simulink model "ironCub"  (Simulink 8.6)
settings: Solver=FixedStepAuto  StartTime=0.0  StopTime=config.simulationTime  FixedStep=config.Ts  RelTol=1e-3
InitFcn:
  | cd(fileparts(which(bdroot)));
  | initIronCub;
StopFcn:
  | visualizer_demo(time.Data,state.Data,config,desired_x_dx_ddx_dddx_CoM,jetsIntensitiesByWeight);
values from neighbouring files (symbols this model uses):
  config = struct    [initIronCub.m]
  ROBOT_DOF = config.ndof    [initIronCub.m]
libraries: WBToolboxLibrary x99
(part 1 of 2)
settings Model: Creator=DanielePucci  LastModifiedBy=DanielePucci
settings DataIOCC: SaveFormat=Dataset  SignalLoggingSaveFormat=Dataset
settings OptimizationCC: ExpressionDepthLimit=128
settings DebuggingCC: UnderspecifiedInitializationDetection=Simplified  MergeDetectMultiDrivingBlocksExec=error  SolverPrmCheckMsg=none  FcnCallInpInsideContextMsg=EnableAllAsError  StateNameClashWarn=none
settings HardwareCC: ProdBitPerPointer=64  ProdLargestAtomicFloat=Float  ProdIntDivRoundTo=Zero  ProdEndianess=LittleEndian  ProdWordSize=64  ProdHWDeviceType=Intel->x86-64 (Windows64)
settings GRTTargetCC: GeneratePreprocessorConditionals=Use local settings  CombineOutputUpdateFcns=on  GRTInterface=off
settings ConfigComp: CovModelRefEnable=off

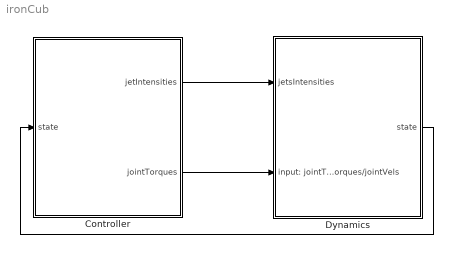
== system ironCub ==
  Controller : Subsystem
  Dynamics : Subsystem
  wires:
  Controller/1(jetIntensities) -> Dynamics/1(jetsIntensities)
  Controller/2(jointTorques) -> Dynamics/2(input: jointTorques/jointVels)
  Dynamics/1(state) -> Controller/1(state)

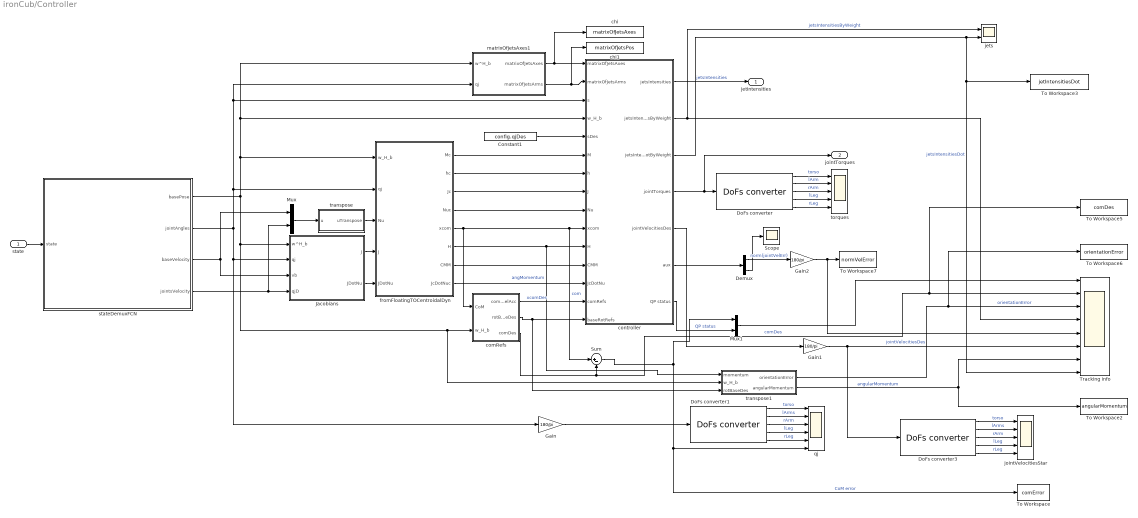
== system ironCub/Controller ==
  state : Inport
  Constant1 : Constant  Value=config.qjDes
  Demux : Demux  Outputs=2
  DoFs converter : WBToolboxLibrary/Utilities/DoFs converter  yarp2WBIOption=From WBI to YARP  robotName=WBT_robotName  localName=WBT_modelName  wbiFile=WBT_wbiFilename  wbiList=WBT_wbiList
  DoFs converter1 : WBToolboxLibrary/Utilities/DoFs converter  yarp2WBIOption=From WBI to YARP  robotName=WBT_robotName  localName=WBT_modelName  wbiFile=WBT_wbiFilename  wbiList=WBT_wbiList
  DoFs converter3 : WBToolboxLibrary/Utilities/DoFs converter  yarp2WBIOption=From WBI to YARP  robotName=WBT_robotName  localName=WBT_modelName  wbiFile=WBT_wbiFilename  wbiList=WBT_wbiList
  Gain : Gain  Gain=180/pi
  Gain1 : Gain  Gain=180/pi
  Gain2 : Gain  Gain=180/pi
  Jacobians : Subsystem
  Mux : Mux  Inputs=2
  Mux1 : Mux  Inputs=2
  Scope : Scope
  Sum : Sum  Inputs=|+-
  To Workspace : ToWorkspace  VariableName=comError  SaveFormat=Timeseries  SampleTime=-1
  To Workspace2 : ToWorkspace  VariableName=angularMomentum  SaveFormat=Timeseries  SampleTime=-1
  To Workspace3 : ToWorkspace  VariableName=jetIntensitiesDot  SaveFormat=Timeseries  SampleTime=-1
  To Workspace5 : ToWorkspace  VariableName=comDes  SaveFormat=Timeseries  SampleTime=-1
  To Workspace6 : ToWorkspace  VariableName=orientationError  SaveFormat=Timeseries  SampleTime=-1
  To Workspace7 : ToWorkspace  VariableName=normVelError  SaveFormat=Timeseries  SampleTime=-1
  Tracking info : Scope  NumInputPorts=8
  chi : ToWorkspace  VariableName=matrixOfJetsAxes  SaveFormat=Timeseries  SampleTime=-1
  chi1 : ToWorkspace  VariableName=matrixOfJetsPos  SaveFormat=Timeseries  SampleTime=-1
  comRefs : Subsystem
  controller : Subsystem
  fromFloatingTOCentroidalDyn : Subsystem
  jets : Scope  NumInputPorts=2
  jointVelocitiesStar : Scope  NumInputPorts=5
  matrixOfJetsAxes1 : Subsystem
  qj : Scope  NumInputPorts=6
  stateDemuxFCN : MATLAB Function  TreatAsAtomicUnit=on
  torques : Scope  NumInputPorts=5
  transpose : MATLAB Function  TreatAsAtomicUnit=on
  transpose1 : MATLAB Function  TreatAsAtomicUnit=on
  jetIntensities : Outport
  jointTorques : Outport  Port=2
  wires:
  state/1 -> stateDemuxFCN/1(state)
  stateDemuxFCN/4(jointsVelocity) -> Mux/2, Jacobians/4(qjD)
  stateDemuxFCN/2(jointAngles) -> Gain/1, Jacobians/2(qj), matrixOfJetsAxes1/2(qj), controller/3(s), fromFloatingTOCentroidalDyn/2(qj)
  stateDemuxFCN/1(basePose) -> controller/4(w_H_b), matrixOfJetsAxes1/1(w^H_b), fromFloatingTOCentroidalDyn/1(w_H_b), transpose1/2(w_H_b), comRefs/2(w_H_b), Jacobians/1(w^H_b)
  Jacobians/1(J) -> fromFloatingTOCentroidalDyn/4(J)
  matrixOfJetsAxes1/1(matrixOfJetsAxes) -> chi/1, controller/1(matrixOfJetsAxes)
  stateDemuxFCN/3(baseVelocity) -> Mux/1, Jacobians/3(vb)
  fromFloatingTOCentroidalDyn/1(Mc) -> controller/6(M)
  fromFloatingTOCentroidalDyn/2("hc ") -> controller/7(h)
  fromFloatingTOCentroidalDyn/3(Jc) -> controller/8(J)
  fromFloatingTOCentroidalDyn/4(Nuc) -> controller/9(Nu)
  fromFloatingTOCentroidalDyn/5(xcom) -> Sum/1, controller/10(xcom), comRefs/1(CoM)  "com"
  controller/4(jointTorques) -> DoFs converter/1, jointTorques/1
  controller/1(jetsIntensities) -> jetIntensities/1  "jetsIntensities"
  Constant1/1 -> controller/5(sDes)
  comRefs/1(comDesPosVelAcc) -> controller/14(comRefs)  "xcomDes"
  Sum/1 -> Mux1/1, qj/6, To Workspace/1  "CoM error"
  DoFs converter1/3 -> qj/3  "rArm"
  DoFs converter1/1 -> qj/1  "torso"
  DoFs converter1/4 -> qj/4  "lLeg"
  DoFs converter1/2 -> qj/2  "lArms"
  DoFs converter1/5 -> qj/5  "rLeg"
  DoFs converter/3 -> torques/3  "rArm"
  DoFs converter/1 -> torques/1  "torso"
  DoFs converter/4 -> torques/4  "lLeg"
  DoFs converter/2 -> torques/2  "lArm"
  DoFs converter/5 -> torques/5  "rLeg"
  Mux/1 -> transpose/1(u)
  transpose/1(uTranspose) -> fromFloatingTOCentroidalDyn/3(Nu)
  Jacobians/2(JDotNu) -> fromFloatingTOCentroidalDyn/5(JDotNu)
  fromFloatingTOCentroidalDyn/8(JcDotNuc) -> controller/13(JcDotNu)
  matrixOfJetsAxes1/2(matrixOfJetsArms) -> chi1/1, controller/2(matrixOfJetsArms)
  fromFloatingTOCentroidalDyn/6(H) -> transpose1/1(momentum), controller/11(H)  "angMomentum"
  fromFloatingTOCentroidalDyn/7(CMM) -> controller/12(CMM)
  Gain/1 -> DoFs converter1/1
  controller/6(aux) -> Demux/1
  Demux/1 -> Gain2/1  "norm(jointVelErr)"
  controller/5(jointVelocitiesDes) -> Gain1/1
  transpose1/1(orientationError) -> To Workspace6/1, Tracking info/3  "orientationError"
  Demux/2 -> Scope/1
  comRefs/2(rotBaseDes) -> transpose1/3(rotBaseDes), controller/15(baseRotRefs)
  comRefs/3(comDes) -> To Workspace5/1, Tracking info/2, Sum/2  "comDes"
  Gain1/1 -> DoFs converter3/1, Tracking info/6  "jointVelocitiesDes"
  controller/3(jetsIntensitiesDotByWeight) -> jets/2, To Workspace3/1, Tracking info/8  "jetsIntensitiesDot"
  Mux1/1 -> Tracking info/1
  controller/7(QP status) -> Mux1/2  "QP status"
  controller/2(jetsIntensitiesByWeight) -> Tracking info/4, jets/1  "jetsIntensitiesByWeight"
  DoFs converter3/3 -> jointVelocitiesStar/3  "rArm"
  DoFs converter3/1 -> jointVelocitiesStar/1  "torso"
  DoFs converter3/4 -> jointVelocitiesStar/4  "lLeg"
  DoFs converter3/2 -> jointVelocitiesStar/2  "lArms"
  DoFs converter3/5 -> jointVelocitiesStar/5  "rLeg"
  transpose1/2(angularMomentum) -> To Workspace2/1, Tracking info/7  "angularMomentum"
  Gain2/1 -> Tracking info/5, To Workspace7/1

== system ironCub/Dynamics ==
  jetsIntensities : Inport
  input: jointTorques/jointVels : Inport  Port=2
  Clock : Clock
  Get Bias Forces : WBToolboxLibrary/wholeBodyModel/Dynamics/Get Bias Forces  robotName=WBT_robotName  localName=WBT_modelName  wbiFile=WBT_wbiFilename  wbiList=WBT_wbiList  explicitGravity=off
  Integrator : Integrator  InitialCondition=config.state0
  Mass Matrix : WBToolboxLibrary/wholeBodyModel/Dynamics/Mass Matrix  robotName=WBT_robotName  localName=WBT_modelName  wbiFile=WBT_wbiFilename  wbiList=WBT_wbiList
  Subsystem : Subsystem  Commented=on
  chi : ToWorkspace  VariableName=state  SaveFormat=Timeseries  SampleTime=-1
  "dyanmicsFCN " : MATLAB Function  TreatAsAtomicUnit=on
  fromStateToForces : Subsystem
  stateDemuxFCN : MATLAB Function  TreatAsAtomicUnit=on
  t : ToWorkspace  VariableName=time  SaveFormat=Timeseries  SampleTime=-1
  state : Outport
  wires:
  "dyanmicsFCN "/1(stateDot) -> Integrator/1
  input: jointTorques/jointVels/1 -> Subsystem/1(input), "dyanmicsFCN "/5(tau)
  stateDemuxFCN/4(jointsVelocity) -> Get Bias Forces/4
  stateDemuxFCN/2(jointAngles) -> Get Bias Forces/2, fromStateToForces/2(jointPosition), Mass Matrix/2
  stateDemuxFCN/1(basePose) -> Get Bias Forces/1, fromStateToForces/1(basePose), Mass Matrix/1
  stateDemuxFCN/3(baseVelocity) -> Get Bias Forces/3
  Mass Matrix/1 -> "dyanmicsFCN "/1(M)
  Get Bias Forces/1 -> "dyanmicsFCN "/2(h)
  jetsIntensities/1 -> fromStateToForces/3(jetsIntensities)
  fromStateToForces/1(J) -> "dyanmicsFCN "/3(J)
  fromStateToForces/2(f) -> "dyanmicsFCN "/4(f)
  Clock/1 -> t/1
  Integrator/1 -> Subsystem/2(state), chi/1, stateDemuxFCN/1(state), "dyanmicsFCN "/6(state), state/1

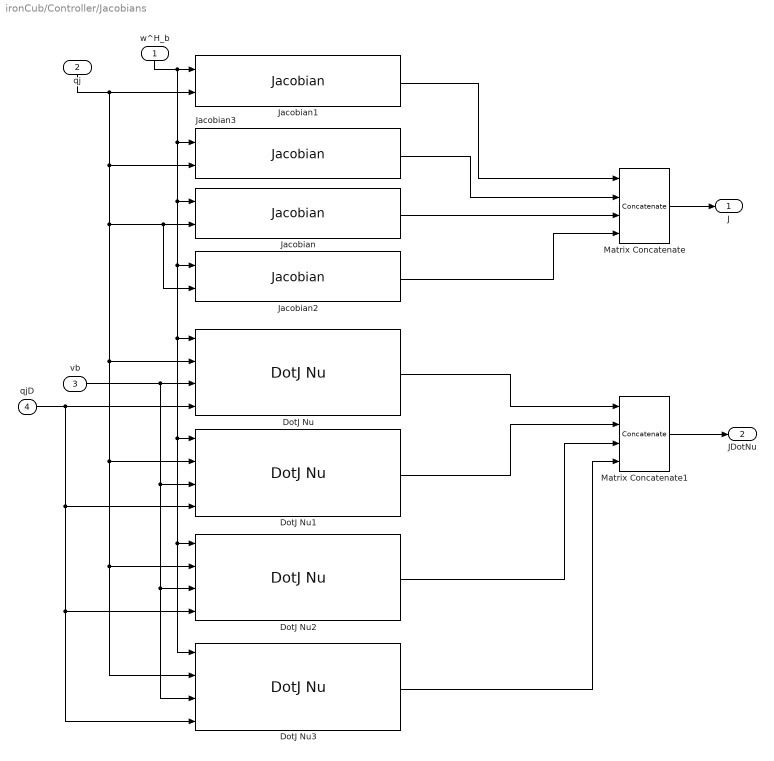
== system ironCub/Controller/Jacobians ==
  w^H_b : Inport
  qj : Inport  Port=2
  vb : Inport  Port=3
  qjD : Inport  Port=4
  DotJ Nu : WBToolboxLibrary/wholeBodyModel/Jacobians/DotJ Nu  frameName='l_hand_dh_frame'  robotName=WBT_robotName  localName=WBT_modelName  wbiFile=WBT_wbiFilename  wbiList=WBT_wbiList
  DotJ Nu1 : WBToolboxLibrary/wholeBodyModel/Jacobians/DotJ Nu  frameName='r_hand_dh_frame'  robotName=WBT_robotName  localName=WBT_modelName  wbiFile=WBT_wbiFilename  wbiList=WBT_wbiList
  DotJ Nu2 : WBToolboxLibrary/wholeBodyModel/Jacobians/DotJ Nu  frameName='l_foot_dh_frame'  robotName=WBT_robotName  localName=WBT_modelName  wbiFile=WBT_wbiFilename  wbiList=WBT_wbiList
  DotJ Nu3 : WBToolboxLibrary/wholeBodyModel/Jacobians/DotJ Nu  frameName='r_foot_dh_frame'  robotName=WBT_robotName  localName=WBT_modelName  wbiFile=WBT_wbiFilename  wbiList=WBT_wbiList
  Jacobian : WBToolboxLibrary/wholeBodyModel/Jacobians/Jacobian  frameName='l_foot_dh_frame'  robotName=WBT_robotName  localName=WBT_modelName  wbiFile=WBT_wbiFilename  wbiList=WBT_wbiList
  Jacobian1 : WBToolboxLibrary/wholeBodyModel/Jacobians/Jacobian  frameName='l_hand_dh_frame'  robotName=WBT_robotName  localName=WBT_modelName  wbiFile=WBT_wbiFilename  wbiList=WBT_wbiList
  Jacobian2 : WBToolboxLibrary/wholeBodyModel/Jacobians/Jacobian  frameName='r_foot_dh_frame'  robotName=WBT_robotName  localName=WBT_modelName  wbiFile=WBT_wbiFilename  wbiList=WBT_wbiList
  Jacobian3 : WBToolboxLibrary/wholeBodyModel/Jacobians/Jacobian  frameName='r_hand_dh_frame'  robotName=WBT_robotName  localName=WBT_modelName  wbiFile=WBT_wbiFilename  wbiList=WBT_wbiList
  Matrix Concatenate : Concatenate  NumInputs=4  Mode=Multidimensional array
  Matrix Concatenate1 : Concatenate  NumInputs=4  Mode=Multidimensional array
  J : Outport
  JDotNu : Outport  Port=2
  wires:
  Matrix Concatenate/1 -> J/1
  w^H_b/1 -> Jacobian1/1, Jacobian3/1, DotJ Nu3/1, DotJ Nu2/1, DotJ Nu1/1, DotJ Nu/1, Jacobian2/1, Jacobian/1
  Jacobian1/1 -> Matrix Concatenate/1
  Jacobian3/1 -> Matrix Concatenate/2
  Jacobian/1 -> Matrix Concatenate/3
  Jacobian2/1 -> Matrix Concatenate/4
  qj/1 -> Jacobian1/2, Jacobian3/2, DotJ Nu3/2, DotJ Nu2/2, DotJ Nu1/2, DotJ Nu/2, Jacobian2/2, Jacobian/2
  vb/1 -> DotJ Nu3/3, DotJ Nu2/3, DotJ Nu1/3, DotJ Nu/3
  qjD/1 -> DotJ Nu3/4, DotJ Nu2/4, DotJ Nu1/4, DotJ Nu/4
  DotJ Nu/1 -> Matrix Concatenate1/1
  DotJ Nu1/1 -> Matrix Concatenate1/2
  DotJ Nu2/1 -> Matrix Concatenate1/3
  DotJ Nu3/1 -> Matrix Concatenate1/4
  Matrix Concatenate1/1 -> JDotNu/1

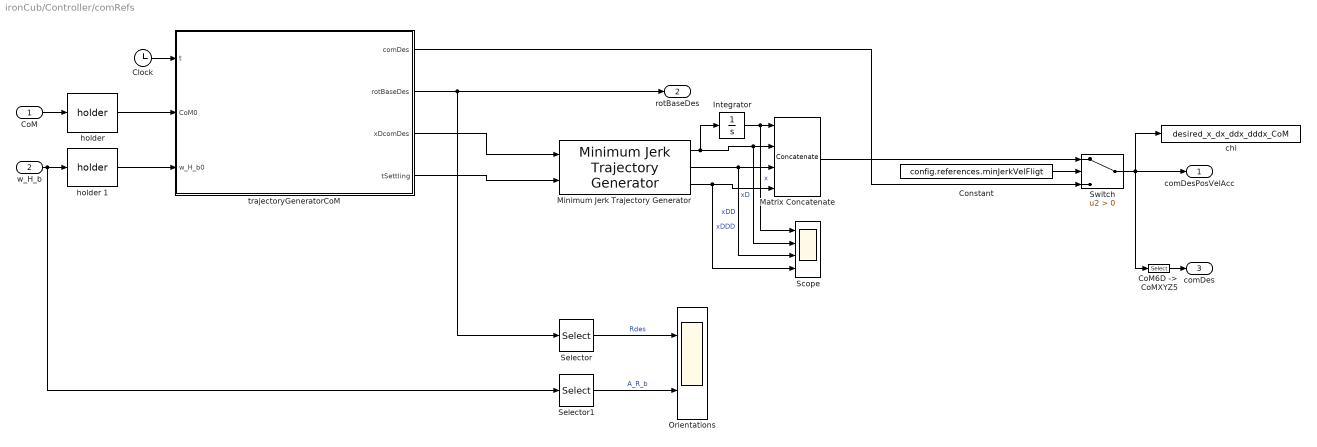
== system ironCub/Controller/comRefs ==
  CoM : Inport
  w_H_b : Inport  Port=2
  Clock : Clock
  "CoM6D ->  CoMXYZ5" : Selector  NumberOfDimensions=2  InputPortWidth=7  IndexOptions=Index vector (dialog),Index vector (dialog)  Indices=[1 2 3],[1]  OutputSizes=1,1
  Constant : Constant  Value=config.references.minJerkVelFligt
  Integrator : Integrator  InitialCondition=config.references.minJerkVel.comDes0
  Matrix Concatenate : Concatenate  NumInputs=4  Mode=Multidimensional array  ConcatenateDimension=2
  Minimum Jerk Trajectory Generator : WBToolboxLibrary/Utilities/Minimum Jerk Trajectory Generator  externalSettlingTime=on  settlingTime=3  sampleTime=config.Ts  resetOnSettlingTime=off  firstDerivatives=on  secondDerivatives=on  explicitInitialValue=off
  Orientations : Scope  NumInputPorts=2
  Scope : Scope  NumInputPorts=4
  Selector : Selector  NumberOfDimensions=2  InputPortWidth=3  IndexOptions=Index vector (dialog),Index vector (dialog)  Indices=[1 2 3],[1 2 3]  OutputSizes=1,1
  Selector1 : Selector  NumberOfDimensions=2  InputPortWidth=3  IndexOptions=Index vector (dialog),Index vector (dialog)  Indices=[1 2 3],[1 2 3]  OutputSizes=1,1
  Switch : Switch  Criteria=u2 > Threshold
  chi : ToWorkspace  VariableName=desired_x_dx_ddx_dddx_CoM  SaveFormat=Timeseries  SampleTime=-1
  "holder " : WBToolboxLibrary/Utilities/holder 
  holder 1 : WBToolboxLibrary/Utilities/holder 
  trajectoryGeneratorCoM : MATLAB Function  TreatAsAtomicUnit=on
  comDesPosVelAcc : Outport
  rotBaseDes : Outport  Port=2
  comDes : Outport  Port=3
  wires:
  Clock/1 -> trajectoryGeneratorCoM/1(t)
  trajectoryGeneratorCoM/1(comDes) -> Switch/3
  CoM/1 -> "holder "/1
  "holder "/1 -> trajectoryGeneratorCoM/2(CoM0)
  w_H_b/1 -> Selector1/1, holder 1/1
  trajectoryGeneratorCoM/2(rotBaseDes) -> Selector/1, rotBaseDes/1
  holder 1/1 -> trajectoryGeneratorCoM/3(w_H_b0)
  trajectoryGeneratorCoM/3(xDcomDes) -> Minimum Jerk Trajectory Generator/1
  trajectoryGeneratorCoM/4(tSettling) -> Minimum Jerk Trajectory Generator/2
  Integrator/1 -> Scope/1, Matrix Concatenate/1  "x"
  Minimum Jerk Trajectory Generator/1 -> Integrator/1, Scope/2, Matrix Concatenate/2  "xD"
  Minimum Jerk Trajectory Generator/2 -> Scope/3, Matrix Concatenate/3  "xDD"
  Minimum Jerk Trajectory Generator/3 -> Scope/4, Matrix Concatenate/4  "xDDD"
  Matrix Concatenate/1 -> Switch/1
  Switch/1 -> "CoM6D ->  CoMXYZ5"/1, chi/1, comDesPosVelAcc/1
  Constant/1 -> Switch/2
  "CoM6D ->  CoMXYZ5"/1 -> comDes/1
  Selector/1 -> Orientations/1  "Rdes"
  Selector1/1 -> Orientations/2  "A_R_b"

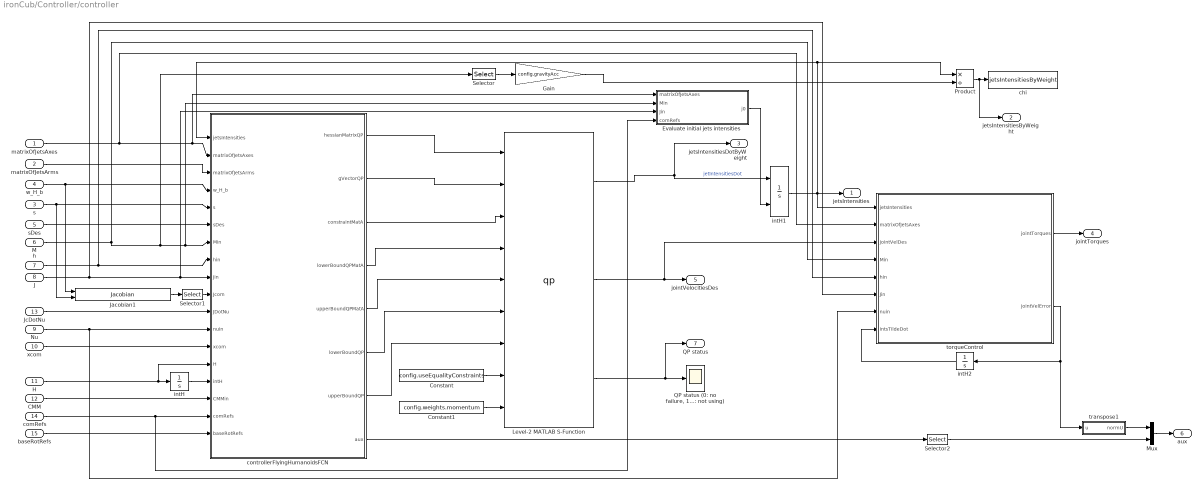
== system ironCub/Controller/controller ==
  matrixOfJetsAxes : Inport
  matrixOfJetsArms : Inport  Port=2
  s : Inport  Port=3
  w_H_b : Inport  Port=4
  sDes : Inport  Port=5
  M : Inport  Port=6
  h : Inport  Port=7
  J : Inport  Port=8
  Nu : Inport  Port=9
  xcom : Inport  Port=10
  H : Inport  Port=11
  CMM : Inport  Port=12
  JcDotNu : Inport  Port=13
  comRefs : Inport  Port=14
  baseRotRefs : Inport  Port=15
  Constant : Constant  Value=config.useEqualityConstraints
  Constant1 : Constant  Value=config.weights.momentum
  Evaluate initial jets intensities : MATLAB Function  TreatAsAtomicUnit=on
  Gain : Gain  Gain=config.gravityAcc
  Jacobian1 : WBToolboxLibrary/wholeBodyModel/Jacobians/Jacobian  frameName='com'  robotName=WBT_robotName  localName=WBT_modelName  wbiFile=WBT_wbiFilename  wbiList=WBT_wbiList
  Level-2 MATLAB S-Function : M-S-Function  FunctionName=qp  Parameters=config.ndof  mask{ndof=config.ndof}
      mask prompts: ndof "Robt degrees of freedom"
      mask Display: disp('QP')
  Mux : Mux  Inputs=2
  Product : Product  Inputs=*/
  "QP status (0: no failure, 1: not using)" : Scope
  Selector : Selector  NumberOfDimensions=2  InputPortWidth=3  IndexOptions=Index vector (dialog),Index vector (dialog)  Indices=1,1  OutputSizes=1,1
  Selector1 : Selector  NumberOfDimensions=2  InputPortWidth=3  IndexOptions=Index vector (dialog),Index vector (dialog)  Indices=[1 2 3],[1:config.ndof+6]  OutputSizes=1,1
  Selector2 : Selector  InputPortWidth=2  IndexOptions=Index vector (dialog)  Indices=[2]  OutputSizes=1
  chi : ToWorkspace  VariableName=jetsIntensitiesByWeight  SaveFormat=Timeseries  SampleTime=-1
  controllerFlyingHumanoidsFCN : MATLAB Function  TreatAsAtomicUnit=on
  intH : Integrator  InitialCondition=zeros(6,1)
  intH1 : Integrator  InitialConditionSource=external  InitialCondition=config.jetsIntensities0
  intH2 : Integrator  InitialCondition=zeros(config.ndof,1)
  torqueControl : MATLAB Function  TreatAsAtomicUnit=on
  transpose1 : MATLAB Function  TreatAsAtomicUnit=on
  jetsIntensities : Outport
  jetsIntensitiesByWeight : Outport  Port=2
  jetsIntensitiesDotByWeight : Outport  Port=3
  jointTorques : Outport  Port=4
  jointVelocitiesDes : Outport  Port=5
  aux : Outport  Port=6
  QP status : Outport  Port=7
  wires:
  matrixOfJetsAxes/1 -> controllerFlyingHumanoidsFCN/2(matrixOfJetsAxes), Evaluate initial jets intensities/1(matrixOfJetsAxes), torqueControl/2(matrixOfJetsAxes)
  M/1 -> Evaluate initial jets intensities/2(Min), controllerFlyingHumanoidsFCN/7(Min), Selector/1, torqueControl/4(Min)
  h/1 -> torqueControl/5(hin), controllerFlyingHumanoidsFCN/8(hin)
  J/1 -> Evaluate initial jets intensities/3(Jin), controllerFlyingHumanoidsFCN/9(Jin), torqueControl/6(Jin)
  Nu/1 -> torqueControl/7(nuin), controllerFlyingHumanoidsFCN/12(nuin)
  xcom/1 -> controllerFlyingHumanoidsFCN/13(xcom)
  comRefs/1 -> Evaluate initial jets intensities/4(comRefs), controllerFlyingHumanoidsFCN/17(comRefs)
  s/1 -> controllerFlyingHumanoidsFCN/5(s), Jacobian1/2
  sDes/1 -> controllerFlyingHumanoidsFCN/6(sDes)
  H/1 -> controllerFlyingHumanoidsFCN/14(H), intH/1
  JcDotNu/1 -> controllerFlyingHumanoidsFCN/11(JDotNu)
  matrixOfJetsArms/1 -> controllerFlyingHumanoidsFCN/3(matrixOfJetsArms)
  intH/1 -> controllerFlyingHumanoidsFCN/15(intH)
  CMM/1 -> controllerFlyingHumanoidsFCN/16(CMMin)
  Selector/1 -> Gain/1
  Product/1 -> jetsIntensitiesByWeight/1, chi/1
  Gain/1 -> Product/2
  intH1/1 -> controllerFlyingHumanoidsFCN/1(jetsIntensities), Product/1, torqueControl/1(jetsIntensities), jetsIntensities/1
  controllerFlyingHumanoidsFCN/8(aux) -> Selector2/1
  Evaluate initial jets intensities/1(j0) -> intH1/2
  baseRotRefs/1 -> controllerFlyingHumanoidsFCN/18(baseRotRefs)
  w_H_b/1 -> controllerFlyingHumanoidsFCN/4(w_H_b), Jacobian1/1
  torqueControl/1(jointTorques) -> jointTorques/1
  Level-2 MATLAB S-Function/1 -> jetsIntensitiesDotByWeight/1, intH1/1  "jetIntensitiesDot"
  controllerFlyingHumanoidsFCN/1(hessianMatrixQP) -> Level-2 MATLAB S-Function/1
  controllerFlyingHumanoidsFCN/2(gVectorQP) -> Level-2 MATLAB S-Function/2
  controllerFlyingHumanoidsFCN/3(constraintMatA) -> Level-2 MATLAB S-Function/3
  intH2/1 -> torqueControl/8(intsTildeDot)
  torqueControl/2(jointVelError) -> transpose1/1(u), intH2/1
  Level-2 MATLAB S-Function/2 -> torqueControl/3(jointVelDes), jointVelocitiesDes/1
  controllerFlyingHumanoidsFCN/6(lowerBoundQP) -> Level-2 MATLAB S-Function/6
  controllerFlyingHumanoidsFCN/7(upperBoundQP) -> Level-2 MATLAB S-Function/7
  Level-2 MATLAB S-Function/3 -> "QP status (0: no failure, 1: not using)"/1, QP status/1
  controllerFlyingHumanoidsFCN/4(lowerBoundQPMatA) -> Level-2 MATLAB S-Function/4
  controllerFlyingHumanoidsFCN/5(upperBoundQPMatA) -> Level-2 MATLAB S-Function/5
  Constant/1 -> Level-2 MATLAB S-Function/8
  Constant1/1 -> Level-2 MATLAB S-Function/9
  Jacobian1/1 -> Selector1/1
  Selector1/1 -> controllerFlyingHumanoidsFCN/10(Jcom)
  Mux/1 -> aux/1
  Selector2/1 -> Mux/2
  transpose1/1(normU) -> Mux/1

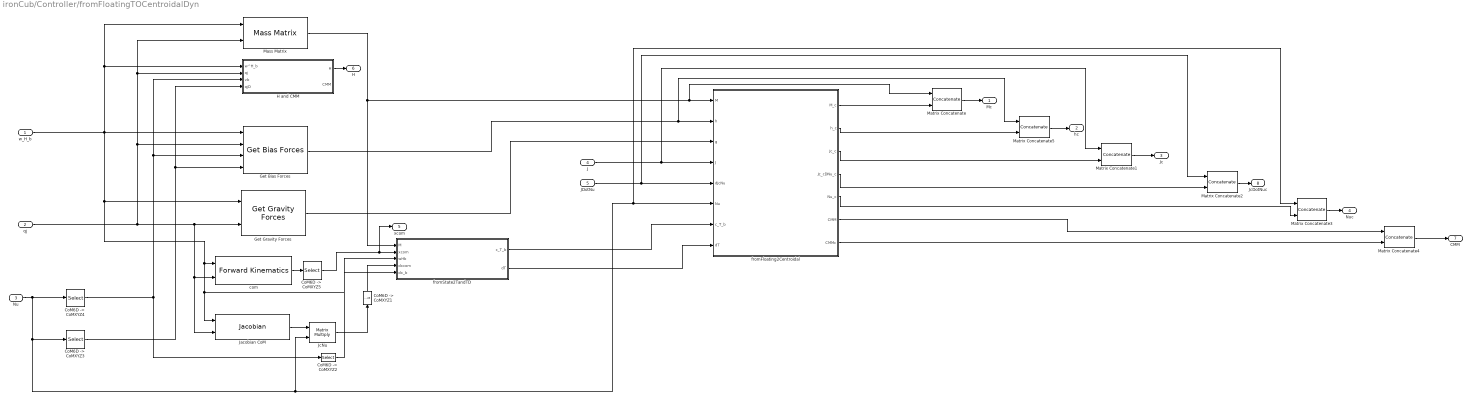
== system ironCub/Controller/fromFloatingTOCentroidalDyn ==
  w_H_b : Inport
  qj : Inport  Port=2
  Nu : Inport  Port=3
  J : Inport  Port=4
  JDotNu : Inport  Port=5
  "CoM6D ->  CoMXYZ1" : Selector  InputPortWidth=6  IndexOptions=Index vector (dialog)  Indices=[1 2 3]  OutputSizes=1
  "CoM6D ->  CoMXYZ2" : Selector  InputPortWidth=6  IndexOptions=Index vector (dialog)  Indices=[1 2 3]  OutputSizes=1
  "CoM6D ->  CoMXYZ3" : Selector  InputPortWidth=6+config.ndof  IndexOptions=Index vector (dialog)  Indices=[7:6+config.ndof]  OutputSizes=1
  "CoM6D ->  CoMXYZ4" : Selector  InputPortWidth=6+config.ndof  IndexOptions=Index vector (dialog)  Indices=[1 2 3 4 5 6]  OutputSizes=1
  "CoM6D ->  CoMXYZ5" : Selector  NumberOfDimensions=2  InputPortWidth=7  IndexOptions=Index vector (dialog),Index vector (dialog)  Indices=[1 2 3],[4]  OutputSizes=1,1
  Get Bias Forces : WBToolboxLibrary/wholeBodyModel/Dynamics/Get Bias Forces  robotName=WBT_robotName  localName=WBT_modelName  wbiFile=WBT_wbiFilename  wbiList=WBT_wbiList  explicitGravity=off
  Get Gravity Forces : WBToolboxLibrary/wholeBodyModel/Dynamics/Get Gravity Forces  robotName=WBT_robotName  localName=WBT_modelName  wbiFile=WBT_wbiFilename  wbiList=WBT_wbiList  explicitGravity=off
  H and CMM : Subsystem
  Jacobian CoM : WBToolboxLibrary/wholeBodyModel/Jacobians/Jacobian  frameName='com'  robotName=WBT_robotName  localName=WBT_modelName  wbiFile=WBT_wbiFilename  wbiList=WBT_wbiList
  JcNu : Product  Multiplication=Matrix(*)
  Mass Matrix : WBToolboxLibrary/wholeBodyModel/Dynamics/Mass Matrix  robotName=WBT_robotName  localName=WBT_modelName  wbiFile=WBT_wbiFilename  wbiList=WBT_wbiList
  Matrix Concatenate{,2..3,5} (4 alike) : Concatenate  Mode=Multidimensional array  ConcatenateDimension=2
  Matrix Concatenate1 : Concatenate  Mode=Multidimensional array
  Matrix Concatenate4 : Concatenate  Mode=Multidimensional array
  com : WBToolboxLibrary/wholeBodyModel/Kinematics/Forward Kinematics  frameName='com'  robotName=WBT_robotName  localName=WBT_modelName  wbiFile=WBT_wbiFilename  wbiList=WBT_wbiList
  fromFloating2Centroidal : MATLAB Function  TreatAsAtomicUnit=on
  fromState2TandTD : MATLAB Function  TreatAsAtomicUnit=on
  Mc : Outport
  "hc " : Outport  Port=2
  Jc : Outport  Port=3
  Nuc : Outport  Port=4
  xcom : Outport  Port=5
  H : Outport  Port=6
  CMM : Outport  Port=7
  JcDotNuc : Outport  Port=8
  wires:
  w_H_b/1 -> fromState2TandTD/3(wHb), Jacobian CoM/1, com/1, Get Gravity Forces/1, Get Bias Forces/1, H and CMM/1(w^H_b), Mass Matrix/1
  qj/1 -> Get Bias Forces/2, H and CMM/2(qj), Mass Matrix/2, Jacobian CoM/2, com/2, Get Gravity Forces/2
  "CoM6D ->  CoMXYZ4"/1 -> "CoM6D ->  CoMXYZ2"/1, H and CMM/3(vb), Get Bias Forces/3
  "CoM6D ->  CoMXYZ3"/1 -> H and CMM/4(qjD), Get Bias Forces/4
  Mass Matrix/1 -> fromState2TandTD/1(M), Matrix Concatenate/1, fromFloating2Centroidal/1(M)
  Get Bias Forces/1 -> Matrix Concatenate5/1, fromFloating2Centroidal/2(h)
  Get Gravity Forces/1 -> fromFloating2Centroidal/3(g)
  J/1 -> Matrix Concatenate1/1, fromFloating2Centroidal/4(J)
  JDotNu/1 -> Matrix Concatenate2/1, fromFloating2Centroidal/5(dJcNu)
  com/1 -> "CoM6D ->  CoMXYZ5"/1
  "CoM6D ->  CoMXYZ5"/1 -> xcom/1, fromState2TandTD/2(xcom)
  Jacobian CoM/1 -> JcNu/1
  JcNu/1 -> "CoM6D ->  CoMXYZ1"/1
  "CoM6D ->  CoMXYZ1"/1 -> fromState2TandTD/4(dxcom)
  fromState2TandTD/1(c_T_b) -> fromFloating2Centroidal/7(c_T_b)
  fromState2TandTD/2(dT) -> fromFloating2Centroidal/8(dT)
  "CoM6D ->  CoMXYZ2"/1 -> fromState2TandTD/5(dx_b)
  Nu/1 -> JcNu/2, Matrix Concatenate3/1, fromFloating2Centroidal/6(Nu), "CoM6D ->  CoMXYZ3"/1, "CoM6D ->  CoMXYZ4"/1
  H and CMM/1(H) -> H/1
  Matrix Concatenate/1 -> Mc/1
  fromFloating2Centroidal/1(M_c) -> Matrix Concatenate/2
  fromFloating2Centroidal/2(h_c) -> Matrix Concatenate5/2
  Matrix Concatenate5/1 -> "hc "/1
  Matrix Concatenate1/1 -> Jc/1
  fromFloating2Centroidal/3(Jc_c) -> Matrix Concatenate1/2
  Matrix Concatenate2/1 -> JcDotNuc/1
  fromFloating2Centroidal/4(Jc_cDNu_c) -> Matrix Concatenate2/2
  Matrix Concatenate3/1 -> Nuc/1
  fromFloating2Centroidal/5(Nu_c) -> Matrix Concatenate3/2
  Matrix Concatenate4/1 -> CMM/1
  fromFloating2Centroidal/7(CMMc) -> Matrix Concatenate4/2
  fromFloating2Centroidal/6(CMM) -> Matrix Concatenate4/1

== system ironCub/Controller/matrixOfJetsAxes1 ==
  w^H_b : Inport
  qj : Inport  Port=2
  "CoM6D ->  CoMXYZ5" : Selector  NumberOfDimensions=2  InputPortWidth=7  IndexOptions=Index vector (dialog),Index vector (dialog)  Indices=[1 2 3],[4]  OutputSizes=1,1
  Forward Kinematics : WBToolboxLibrary/wholeBodyModel/Kinematics/Forward Kinematics  frameName='l_foot_dh_frame'  robotName=WBT_robotName  localName=WBT_modelName  wbiFile=WBT_wbiFilename  wbiList=WBT_wbiList
  Forward Kinematics1 : WBToolboxLibrary/wholeBodyModel/Kinematics/Forward Kinematics  frameName='r_foot_dh_frame'  robotName=WBT_robotName  localName=WBT_modelName  wbiFile=WBT_wbiFilename  wbiList=WBT_wbiList
  Forward Kinematics2 : WBToolboxLibrary/wholeBodyModel/Kinematics/Forward Kinematics  frameName='l_hand_dh_frame'  robotName=WBT_robotName  localName=WBT_modelName  wbiFile=WBT_wbiFilename  wbiList=WBT_wbiList
  Forward Kinematics3 : WBToolboxLibrary/wholeBodyModel/Kinematics/Forward Kinematics  frameName='r_hand_dh_frame'  robotName=WBT_robotName  localName=WBT_modelName  wbiFile=WBT_wbiFilename  wbiList=WBT_wbiList
  com : WBToolboxLibrary/wholeBodyModel/Kinematics/Forward Kinematics  frameName='com'  robotName=WBT_robotName  localName=WBT_modelName  wbiFile=WBT_wbiFilename  wbiList=WBT_wbiList
  stateDemuxFCN : MATLAB Function  TreatAsAtomicUnit=on
  matrixOfJetsAxes : Outport
  matrixOfJetsArms : Outport  Port=2
  wires:
  w^H_b/1 -> com/1, Forward Kinematics1/1, Forward Kinematics/1, Forward Kinematics3/1, Forward Kinematics2/1
  Forward Kinematics3/1 -> stateDemuxFCN/2(w_H_J2)
  qj/1 -> com/2, Forward Kinematics1/2, Forward Kinematics/2, Forward Kinematics3/2, Forward Kinematics2/2
  Forward Kinematics2/1 -> stateDemuxFCN/1(w_H_J1)
  Forward Kinematics/1 -> stateDemuxFCN/3(w_H_J3)
  Forward Kinematics1/1 -> stateDemuxFCN/4(w_H_J4)
  stateDemuxFCN/1(matrixOfJetsAxes) -> matrixOfJetsAxes/1
  stateDemuxFCN/2(matrixOfJetsArms) -> matrixOfJetsArms/1
  com/1 -> "CoM6D ->  CoMXYZ5"/1
  "CoM6D ->  CoMXYZ5"/1 -> stateDemuxFCN/5(com)

== system ironCub/Dynamics/Subsystem ==
  input : Inport
  state : Inport  Port=2
  Constant : Constant  Value=config.considerDynamics
  Gain : Gain  Gain=0
  Integrator1 : Integrator  InitialCondition=config.state0
  Mux : Mux
  Scope : Scope
  Switch : Switch  Criteria=u2 > Threshold
  Terminator : Terminator
  kinematicsFCN : MATLAB Function  TreatAsAtomicUnit=on
  stateDemuxFCN1 : MATLAB Function  TreatAsAtomicUnit=on
  wires:
  input/1 -> Gain/1, Mux/4
  state/1 -> Switch/1
  Switch/1 -> kinematicsFCN/2(state)
  Integrator1/1 -> stateDemuxFCN1/1(state)
  stateDemuxFCN1/4(jointsVelocity) -> Terminator/1
  stateDemuxFCN1/1(basePose) -> Mux/1
  stateDemuxFCN1/2(jointAngles) -> Mux/2
  stateDemuxFCN1/3(baseVelocity) -> Mux/3
  Mux/1 -> Switch/3, Scope/1
  Constant/1 -> Switch/2
  kinematicsFCN/1(stateDot) -> Integrator1/1
  Gain/1 -> kinematicsFCN/1(jointVels)

== system ironCub/Dynamics/fromStateToForces ==
  basePose : Inport
  jointPosition : Inport  Port=2
  jetsIntensities : Inport  Port=3
  Jacobians : Subsystem
  Terminator : Terminator
  fromJetsIntensitiesToForces : MATLAB Function  TreatAsAtomicUnit=on
  matrixOfJetsAxes : Subsystem
  J : Outport
  f : Outport  Port=2
  wires:
  jointPosition/1 -> matrixOfJetsAxes/2(qj), Jacobians/2(qj)
  basePose/1 -> matrixOfJetsAxes/1(w^H_b), Jacobians/1(w^H_b)
  Jacobians/1(J) -> J/1
  fromJetsIntensitiesToForces/1(f) -> f/1
  jetsIntensities/1 -> fromJetsIntensitiesToForces/2(jetsIntensities)
  matrixOfJetsAxes/1(matrixOfJetsAxes) -> fromJetsIntensitiesToForces/1(matrixOfJetsAxes)
  matrixOfJetsAxes/2(matrixOfJetsArms) -> Terminator/1

== system ironCub/Controller/fromFloatingTOCentroidalDyn/H and CMM ==
  w^H_b : Inport
  qj : Inport  Port=2
  vb : Inport  Port=3
  qjD : Inport  Port=4
  Centroidal Momentum : WBToolboxLibrary/wholeBodyModel/Dynamics/Centroidal Momentum  robotName=WBT_robotName  localName=WBT_modelName  wbiFile=WBT_wbiFilename  wbiList=WBT_wbiList
  "Centroidal Momentum Matrix " : Subsystem
  centroidalMomentumMatrixGabry : Subsystem
  H : Outport
  CMM : Outport  Port=2
  wires:
  vb/1 -> Centroidal Momentum/3
  Centroidal Momentum/1 -> H/1
  w^H_b/1 -> centroidalMomentumMatrixGabry/1(W_H_b), "Centroidal Momentum Matrix "/1(w^H_b), Centroidal Momentum/1
  qj/1 -> centroidalMomentumMatrixGabry/2(qj), "Centroidal Momentum Matrix "/2(qj), Centroidal Momentum/2
  qjD/1 -> Centroidal Momentum/4
  "Centroidal Momentum Matrix "/1(CMM) -> CMM/1

== system ironCub/Dynamics/fromStateToForces/Jacobians ==
  w^H_b : Inport
  qj : Inport  Port=2
  Jacobian : WBToolboxLibrary/wholeBodyModel/Jacobians/Jacobian  frameName='l_foot_dh_frame'  robotName=WBT_robotName  localName=WBT_modelName  wbiFile=WBT_wbiFilename  wbiList=WBT_wbiList
  Jacobian1 : WBToolboxLibrary/wholeBodyModel/Jacobians/Jacobian  frameName='l_hand_dh_frame'  robotName=WBT_robotName  localName=WBT_modelName  wbiFile=WBT_wbiFilename  wbiList=WBT_wbiList
  Jacobian2 : WBToolboxLibrary/wholeBodyModel/Jacobians/Jacobian  frameName='r_foot_dh_frame'  robotName=WBT_robotName  localName=WBT_modelName  wbiFile=WBT_wbiFilename  wbiList=WBT_wbiList
  Jacobian3 : WBToolboxLibrary/wholeBodyModel/Jacobians/Jacobian  frameName='r_hand_dh_frame'  robotName=WBT_robotName  localName=WBT_modelName  wbiFile=WBT_wbiFilename  wbiList=WBT_wbiList
  Matrix Concatenate : Concatenate  NumInputs=4  Mode=Multidimensional array
  Selector{,1..3} (4 alike) : Selector  NumberOfDimensions=2  InputPortWidth=3  IndexOptions=Index vector (dialog),Index vector (dialog)  Indices=[1 2 3],[1:config.ndof+6]  OutputSizes=1,1
  J : Outport
  wires:
  Matrix Concatenate/1 -> J/1
  Jacobian/1 -> Selector/1
  Jacobian2/1 -> Selector1/1
  w^H_b/1 -> Jacobian1/1, Jacobian3/1, Jacobian2/1, Jacobian/1
  qj/1 -> Jacobian1/2, Jacobian3/2, Jacobian2/2, Jacobian/2
  Jacobian1/1 -> Selector2/1
  Jacobian3/1 -> Selector3/1
  Selector2/1 -> Matrix Concatenate/1
  Selector3/1 -> Matrix Concatenate/2
  Selector/1 -> Matrix Concatenate/3
  Selector1/1 -> Matrix Concatenate/4

== system ironCub/Dynamics/fromStateToForces/matrixOfJetsAxes ==
  w^H_b : Inport
  qj : Inport  Port=2
  "CoM6D ->  CoMXYZ5" : Selector  NumberOfDimensions=2  InputPortWidth=7  IndexOptions=Index vector (dialog),Index vector (dialog)  Indices=[1 2 3],[4]  OutputSizes=1,1
  Forward Kinematics : WBToolboxLibrary/wholeBodyModel/Kinematics/Forward Kinematics  frameName='l_foot_dh_frame'  robotName=WBT_robotName  localName=WBT_modelName  wbiFile=WBT_wbiFilename  wbiList=WBT_wbiList
  Forward Kinematics1 : WBToolboxLibrary/wholeBodyModel/Kinematics/Forward Kinematics  frameName='r_foot_dh_frame'  robotName=WBT_robotName  localName=WBT_modelName  wbiFile=WBT_wbiFilename  wbiList=WBT_wbiList
  Forward Kinematics2 : WBToolboxLibrary/wholeBodyModel/Kinematics/Forward Kinematics  frameName='l_hand_dh_frame'  robotName=WBT_robotName  localName=WBT_modelName  wbiFile=WBT_wbiFilename  wbiList=WBT_wbiList
  Forward Kinematics3 : WBToolboxLibrary/wholeBodyModel/Kinematics/Forward Kinematics  frameName='r_hand_dh_frame'  robotName=WBT_robotName  localName=WBT_modelName  wbiFile=WBT_wbiFilename  wbiList=WBT_wbiList
  com : WBToolboxLibrary/wholeBodyModel/Kinematics/Forward Kinematics  frameName='com'  robotName=WBT_robotName  localName=WBT_modelName  wbiFile=WBT_wbiFilename  wbiList=WBT_wbiList
  stateDemuxFCN : MATLAB Function  TreatAsAtomicUnit=on
  matrixOfJetsAxes : Outport
  matrixOfJetsArms : Outport  Port=2
  wires:
  w^H_b/1 -> com/1, Forward Kinematics1/1, Forward Kinematics/1, Forward Kinematics3/1, Forward Kinematics2/1
  Forward Kinematics3/1 -> stateDemuxFCN/2(w_H_J2)
  qj/1 -> com/2, Forward Kinematics1/2, Forward Kinematics/2, Forward Kinematics3/2, Forward Kinematics2/2
  Forward Kinematics2/1 -> stateDemuxFCN/1(w_H_J1)
  Forward Kinematics/1 -> stateDemuxFCN/3(w_H_J3)
  Forward Kinematics1/1 -> stateDemuxFCN/4(w_H_J4)
  stateDemuxFCN/1(matrixOfJetsAxes) -> matrixOfJetsAxes/1
  stateDemuxFCN/2(matrixOfJetsArms) -> matrixOfJetsArms/1
  com/1 -> "CoM6D ->  CoMXYZ5"/1
  "CoM6D ->  CoMXYZ5"/1 -> stateDemuxFCN/5(com)

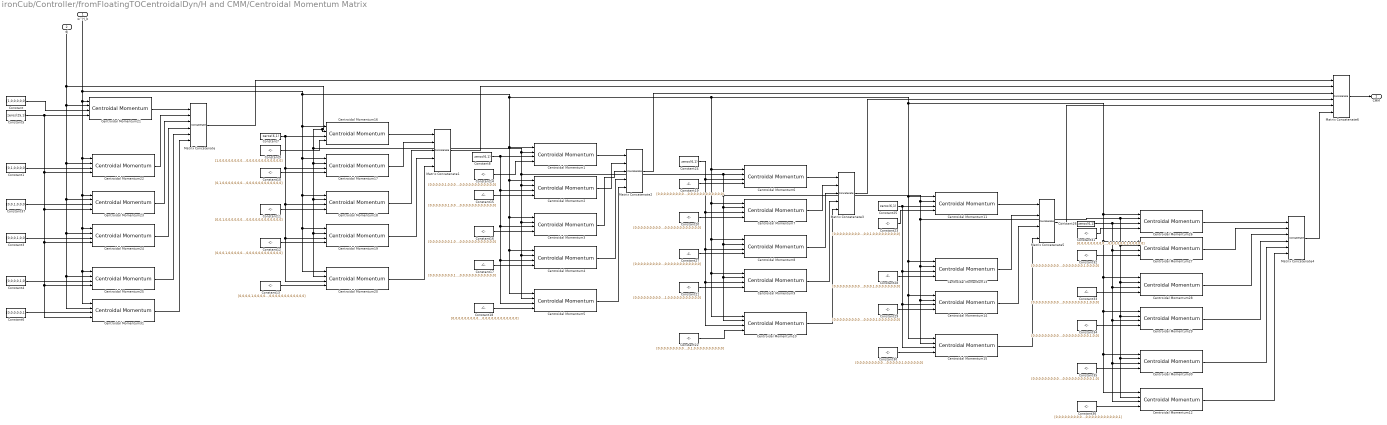
== system ironCub/Controller/fromFloatingTOCentroidalDyn/H and CMM/Centroidal Momentum Matrix  ==
  w^H_b : Inport
  qj : Inport  Port=2
  Centroidal Momentum{1..31} (31 alike) : WBToolboxLibrary/wholeBodyModel/Dynamics/Centroidal Momentum  robotName=WBT_robotName  localName=WBT_modelName  wbiFile=WBT_wbiFilename  wbiList=WBT_wbiList
  Constant : Constant  Value=[1,0,0,0,0,0]
  Constant1 : Constant  Value=[0,1,0,0,0,0]
  Constant10 : Constant  Value=[0,1,0,0,0,0,0,0,0,0,0,0,0,0,0,0,0,0,0,0,0,0,0,0,0]
  Constant11 : Constant  Value=[0,0,1,0,0,0,0,0,0,0,0,0,0,0,0,0,0,0,0,0,0,0,0,0,0]
  Constant12 : Constant  Value=[0,0,0,1,0,0,0,0,0,0,0,0,0,0,0,0,0,0,0,0,0,0,0,0,0]
  Constant13 : Constant  Value=[0,0,0,0,1,0,0,0,0,0,0,0,0,0,0,0,0,0,0,0,0,0,0,0,0]
  Constant14 : Constant  Value=[0,0,0,0,0,1,0,0,0,0,0,0,0,0,0,0,0,0,0,0,0,0,0,0,0]
  Constant15 : Constant  Value=[0,0,0,0,0,0,1,0,0,0,0,0,0,0,0,0,0,0,0,0,0,0,0,0,0]
  Constant16 : Constant  Value=[0,0,0,0,0,0,0,1,0,0,0,0,0,0,0,0,0,0,0,0,0,0,0,0,0]
  Constant17 : Constant  Value=[0,0,0,0,0,0,0,0,1,0,0,0,0,0,0,0,0,0,0,0,0,0,0,0,0]
  Constant18 : Constant  Value=[0,0,0,0,0,0,0,0,0,1,0,0,0,0,0,0,0,0,0,0,0,0,0,0,0]
  Constant19 : Constant  Value=[0,0,0,0,0,0,0,0,0,0,1,0,0,0,0,0,0,0,0,0,0,0,0,0,0]
  Constant20 : Constant  Value=[0,0,0,0,0,0,0,0,0,0,0,1,0,0,0,0,0,0,0,0,0,0,0,0,0]
  Constant21 : Constant  Value=[0,0,0,0,0,0,0,0,0,0,0,0,0,1,0,0,0,0,0,0,0,0,0,0,0]
  Constant22 : Constant  Value=[0,0,0,0,0,0,0,0,0,0,0,0,0,0,1,0,0,0,0,0,0,0,0,0,0]
  Constant23 : Constant  Value=[0,0,0,0,0,0,0,0,0,0,0,0,0,0,0,1,0,0,0,0,0,0,0,0,0]
  Constant{7..8,24..26} (5 alike) : Constant  Value=zeros(6,1)
  Constant27 : Constant  Value=[0,0,0,0,0,0,0,0,0,0,0,0,1,0,0,0,0,0,0,0,0,0,0,0,0]
  Constant28 : Constant  Value=[0,0,0,0,0,0,0,0,0,0,0,0,0,0,0,0,1,0,0,0,0,0,0,0,0]
  Constant29 : Constant  Value=[0,0,0,0,0,0,0,0,0,0,0,0,0,0,0,0,0,1,0,0,0,0,0,0,0]
  Constant3 : Constant  Value=[0,0,0,1,0,0]
  Constant30 : Constant  Value=[0,0,0,0,0,0,0,0,0,0,0,0,0,0,0,0,0,0,1,0,0,0,0,0,0]
  Constant31 : Constant  Value=[0,0,0,0,0,0,0,0,0,0,0,0,0,0,0,0,0,0,0,1,0,0,0,0,0]
  Constant32 : Constant  Value=[0,0,0,0,0,0,0,0,0,0,0,0,0,0,0,0,0,0,0,0,1,0,0,0,0]
  Constant33 : Constant  Value=[0,0,0,0,0,0,0,0,0,0,0,0,0,0,0,0,0,0,0,0,0,1,0,0,0]
  Constant34 : Constant  Value=[0,0,0,0,0,0,0,0,0,0,0,0,0,0,0,0,0,0,0,0,0,0,1,0,0]
  Constant35 : Constant  Value=[0,0,0,0,0,0,0,0,0,0,0,0,0,0,0,0,0,0,0,0,0,0,0,1,0]
  Constant36 : Constant  Value=[0,0,0,0,0,0,0,0,0,0,0,0,0,0,0,0,0,0,0,0,0,0,0,0,1]
  Constant37 : Constant  Value=[0,0,1,0,0,0]
  Constant4 : Constant  Value=[0,0,0,0,1,0]
  Constant5 : Constant  Value=zeros(25,1)
  Constant6 : Constant  Value=[0,0,0,0,0,1]
  Constant9 : Constant  Value=[1,0,0,0,0,0,0,0,0,0,0,0,0,0,0,0,0,0,0,0,0,0,0,0,0]
  Matrix Concatenate : Concatenate  NumInputs=6  Mode=Multidimensional array  ConcatenateDimension=2
  Matrix Concatenate1 : Concatenate  NumInputs=5  Mode=Multidimensional array  ConcatenateDimension=2
  Matrix Concatenate2 : Concatenate  NumInputs=5  Mode=Multidimensional array  ConcatenateDimension=2
  Matrix Concatenate3 : Concatenate  NumInputs=5  Mode=Multidimensional array  ConcatenateDimension=2
  Matrix Concatenate4 : Concatenate  NumInputs=6  Mode=Multidimensional array  ConcatenateDimension=2
  Matrix Concatenate5 : Concatenate  NumInputs=4  Mode=Multidimensional array  ConcatenateDimension=2
  Matrix Concatenate6 : Concatenate  NumInputs=6  Mode=Multidimensional array  ConcatenateDimension=2
  CMM : Outport
  wires:
  Centroidal Momentum19/1 -> Matrix Concatenate1/4
  Centroidal Momentum4/1 -> Matrix Concatenate2/4
  Centroidal Momentum25/1 -> Matrix Concatenate/5
  Matrix Concatenate/1 -> Matrix Concatenate6/1
  Centroidal Momentum12/1 -> Matrix Concatenate4/6
  Centroidal Momentum5/1 -> Matrix Concatenate2/5
  Centroidal Momentum23/1 -> Matrix Concatenate/3
  w^H_b/1 -> Centroidal Momentum5/1, Centroidal Momentum4/1, Centroidal Momentum3/1, Centroidal Momentum2/1, Centroidal Momentum1/1, Centroidal Momentum12/1, Centroidal Momentum30/1, Centroidal Momentum29/1, Centroidal Momentum28/1, Centroidal Momentum27/1, Centroidal Momentum26/1, Centroidal Momentum15/1, Centroidal Momentum14/1, Centroidal Momentum13/1, Centroidal Momentum11/1, Centroidal Momentum10/1, Centroidal Momentum9/1, Centroidal Momentum8/1, Centroidal Momentum7/1, Centroidal Momentum6/1, Centroidal Momentum20/1, Centroidal Momentum19/1, Centroidal Momentum18/1, Centroidal Momentum17/1, Centroidal Momentum16/1, Centroidal Momentum31/1, Centroidal Momentum25/1, Centroidal Momentum24/1, Centroidal Momentum23/1, Centroidal Momentum22/1, Centroidal Momentum21/1
  Matrix Concatenate5/1 -> Matrix Concatenate6/5
  Centroidal Momentum3/1 -> Matrix Concatenate2/3
  Centroidal Momentum29/1 -> Matrix Concatenate4/4
  Matrix Concatenate4/1 -> Matrix Concatenate6/6
  Centroidal Momentum24/1 -> Matrix Concatenate/4
  Centroidal Momentum2/1 -> Matrix Concatenate2/2
  Centroidal Momentum1/1 -> Matrix Concatenate2/1
  Matrix Concatenate1/1 -> Matrix Concatenate6/2
  Centroidal Momentum28/1 -> Matrix Concatenate4/3
  Centroidal Momentum15/1 -> Matrix Concatenate5/4
  Centroidal Momentum7/1 -> Matrix Concatenate3/2
  Centroidal Momentum14/1 -> Matrix Concatenate5/3
  Centroidal Momentum26/1 -> Matrix Concatenate4/1
  Centroidal Momentum27/1 -> Matrix Concatenate4/2
  Matrix Concatenate6/1 -> CMM/1
  Centroidal Momentum6/1 -> Matrix Concatenate3/1
  Centroidal Momentum8/1 -> Matrix Concatenate3/3
  Centroidal Momentum20/1 -> Matrix Concatenate1/5
  Centroidal Momentum11/1 -> Matrix Concatenate5/1
  qj/1 -> Centroidal Momentum22/2, Centroidal Momentum23/2, Centroidal Momentum24/2, Centroidal Momentum31/2, Centroidal Momentum25/2, Centroidal Momentum21/2, Centroidal Momentum14/2, Centroidal Momentum15/2, Centroidal Momentum13/2, Centroidal Momentum12/2, Centroidal Momentum30/2, Centroidal Momentum29/2, Centroidal Momentum28/2, Centroidal Momentum27/2, Centroidal Momentum26/2, Centroidal Momentum11/2, Centroidal Momentum10/2, Centroidal Momentum9/2, Centroidal Momentum8/2, Centroidal Momentum7/2, Centroidal Momentum6/2, Centroidal Momentum5/2, Centroidal Momentum4/2, Centroidal Momentum3/2, Centroidal Momentum2/2, Centroidal Momentum1/2, Centroidal Momentum20/2, Centroidal Momentum19/2, Centroidal Momentum18/2, Centroidal Momentum17/2, Centroidal Momentum16/2
  Matrix Concatenate2/1 -> Matrix Concatenate6/3
  Centroidal Momentum31/1 -> Matrix Concatenate/6
  Centroidal Momentum18/1 -> Matrix Concatenate1/3
  Constant36/1 -> Centroidal Momentum12/4
  Constant23/1 -> Centroidal Momentum11/4
  Constant6/1 -> Centroidal Momentum31/3
  Centroidal Momentum10/1 -> Matrix Concatenate3/5
  Constant18/1 -> Centroidal Momentum5/4
  Constant13/1 -> Centroidal Momentum20/4
  Constant/1 -> Centroidal Momentum21/3
  Constant28/1 -> Centroidal Momentum13/4
  Constant29/1 -> Centroidal Momentum14/4
  Constant1/1 -> Centroidal Momentum22/3
  Constant21/1 -> Centroidal Momentum9/4
  Centroidal Momentum16/1 -> Matrix Concatenate1/1
  Constant14/1 -> Centroidal Momentum1/4
  Constant10/1 -> Centroidal Momentum17/4
  Constant31/1 -> Centroidal Momentum26/4
  Constant8/1 -> Centroidal Momentum5/3, Centroidal Momentum4/3, Centroidal Momentum3/3, Centroidal Momentum2/3, Centroidal Momentum1/3
  Constant37/1 -> Centroidal Momentum23/3
  Constant5/1 -> Centroidal Momentum31/4, Centroidal Momentum25/4, Centroidal Momentum24/4, Centroidal Momentum23/4, Centroidal Momentum22/4, Centroidal Momentum21/4
  Constant22/1 -> Centroidal Momentum10/4
  Constant7/1 -> Centroidal Momentum20/3, Centroidal Momentum19/3, Centroidal Momentum18/3, Centroidal Momentum17/3, Centroidal Momentum16/3
  Constant16/1 -> Centroidal Momentum3/4
  Constant35/1 -> Centroidal Momentum30/4
  Constant12/1 -> Centroidal Momentum19/4
  Constant19/1 -> Centroidal Momentum6/4
  Constant11/1 -> Centroidal Momentum18/4
  Constant4/1 -> Centroidal Momentum25/3
  Constant9/1 -> Centroidal Momentum16/4
  Constant3/1 -> Centroidal Momentum24/3
  Constant32/1 -> Centroidal Momentum27/4
  Constant15/1 -> Centroidal Momentum2/4
  Centroidal Momentum13/1 -> Matrix Concatenate5/2
  Constant34/1 -> Centroidal Momentum29/4
  Constant24/1 -> Centroidal Momentum10/3, Centroidal Momentum9/3, Centroidal Momentum8/3, Centroidal Momentum7/3, Centroidal Momentum6/3
  Constant20/1 -> Centroidal Momentum7/4
  Constant25/1 -> Centroidal Momentum11/3, Centroidal Momentum15/3, Centroidal Momentum14/3, Centroidal Momentum13/3
  Centroidal Momentum9/1 -> Matrix Concatenate3/4
  Constant27/1 -> Centroidal Momentum8/4
  Centroidal Momentum17/1 -> Matrix Concatenate1/2
  Constant26/1 -> Centroidal Momentum12/3, Centroidal Momentum30/3, Centroidal Momentum29/3, Centroidal Momentum28/3, Centroidal Momentum27/3, Centroidal Momentum26/3
  Constant17/1 -> Centroidal Momentum4/4
  Constant30/1 -> Centroidal Momentum15/4
  Constant33/1 -> Centroidal Momentum28/4
  Centroidal Momentum30/1 -> Matrix Concatenate4/5
  Matrix Concatenate3/1 -> Matrix Concatenate6/4
  Centroidal Momentum22/1 -> Matrix Concatenate/2
  Centroidal Momentum21/1 -> Matrix Concatenate/1

== system ironCub/Controller/fromFloatingTOCentroidalDyn/H and CMM/centroidalMomentumMatrixGabry ==
  W_H_b : Inport
  qj : Inport  Port=2
  JGbase : Subsystem
  JGjoints : Subsystem
  Matrix Concatenate : Concatenate  Mode=Multidimensional array  ConcatenateDimension=2
  JG : Outport
  wires:
  qj/1 -> JGjoints/1(qj), JGbase/1(qj)
  W_H_b/1 -> JGjoints/2(W_H_b), JGbase/2(W_H_b)
  JGbase/1(JGbase) -> Matrix Concatenate/1
  JGjoints/1(JGjoints) -> Matrix Concatenate/2
  Matrix Concatenate/1 -> JG/1

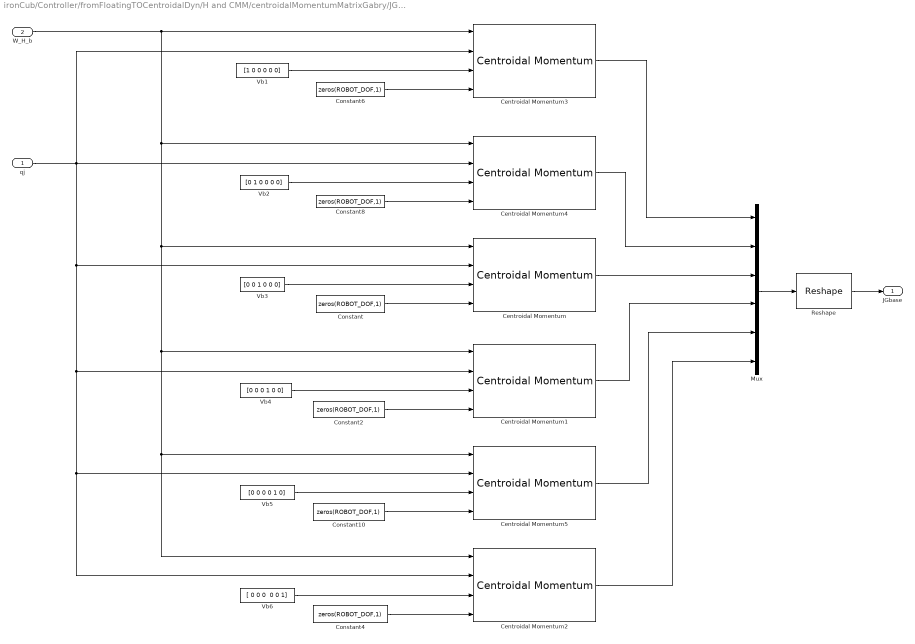
== system ironCub/Controller/fromFloatingTOCentroidalDyn/H and CMM/centroidalMomentumMatrixGabry/JGbase ==
  qj : Inport
  W_H_b : Inport  Port=2
  Centroidal Momentum{,1..5} (6 alike) : WBToolboxLibrary/wholeBodyModel/Dynamics/Centroidal Momentum  robotName=WBT_robotName  localName=WBT_modelName  wbiFile=WBT_wbiFilename  wbiList=WBT_wbiList
  Constant{,2,4,6,8,10} (6 alike) : Constant  Value=zeros(ROBOT_DOF,1)
  Mux : Mux  Inputs=6
  Reshape : Reshape  OutputDimensionality=Customize  OutputDimensions=[6,6]
  Vb1 : Constant  Value=[1 0 0 0 0 0]
  Vb2 : Constant  Value=[0 1 0 0 0 0]
  Vb3 : Constant  Value=[0 0 1 0 0 0]
  Vb4 : Constant  Value=[0 0 0 1 0 0]
  Vb5 : Constant  Value=[0 0 0 0 1 0]
  Vb6 : Constant  Value="[ 0 0 0  0 0 1]"
  JGbase : Outport
  wires:
  Vb1/1 -> Centroidal Momentum3/3
  Vb2/1 -> Centroidal Momentum4/3
  Vb3/1 -> Centroidal Momentum/3
  Vb4/1 -> Centroidal Momentum1/3
  Vb5/1 -> Centroidal Momentum5/3
  Vb6/1 -> Centroidal Momentum2/3
  Constant6/1 -> Centroidal Momentum3/4
  Constant8/1 -> Centroidal Momentum4/4
  Constant/1 -> Centroidal Momentum/4
  Constant2/1 -> Centroidal Momentum1/4
  Constant10/1 -> Centroidal Momentum5/4
  Constant4/1 -> Centroidal Momentum2/4
  qj/1 -> Centroidal Momentum2/2, Centroidal Momentum5/2, Centroidal Momentum1/2, Centroidal Momentum/2, Centroidal Momentum3/2, Centroidal Momentum4/2
  W_H_b/1 -> Centroidal Momentum3/1, Centroidal Momentum2/1, Centroidal Momentum5/1, Centroidal Momentum1/1, Centroidal Momentum/1, Centroidal Momentum4/1
  Centroidal Momentum3/1 -> Mux/1
  Centroidal Momentum4/1 -> Mux/2
  Centroidal Momentum/1 -> Mux/3
  Centroidal Momentum1/1 -> Mux/4
  Centroidal Momentum5/1 -> Mux/5
  Centroidal Momentum2/1 -> Mux/6
  Mux/1 -> Reshape/1
  Reshape/1 -> JGbase/1

== system ironCub/Controller/fromFloatingTOCentroidalDyn/H and CMM/centroidalMomentumMatrixGabry/JGjoints ==
  qj : Inport
  W_H_b : Inport  Port=2
  JGLarm : Subsystem
  JGLleg : Subsystem
  JGRarm : Subsystem
  JGRleg : Subsystem
  JGtorso : Subsystem
  Matrix Concatenate : Concatenate  NumInputs=5  Mode=Multidimensional array  ConcatenateDimension=2
  JGjoints : Outport
  wires:
  qj/1 -> JGRarm/1(qj), JGRleg/1(qj), JGLleg/1(qj), JGLarm/1(qj), JGtorso/1(qj)
  W_H_b/1 -> JGRarm/2(W_H_b), JGRleg/2(W_H_b), JGLleg/2(W_H_b), JGLarm/2(W_H_b), JGtorso/2(W_H_b)
  JGtorso/1(JGtorso) -> Matrix Concatenate/1
  JGLarm/1(JGLarm) -> Matrix Concatenate/2
  JGRarm/1(JGRarm) -> Matrix Concatenate/3
  JGLleg/1(JGLleg) -> Matrix Concatenate/4
  JGRleg/1(JGRleg) -> Matrix Concatenate/5
  Matrix Concatenate/1 -> JGjoints/1

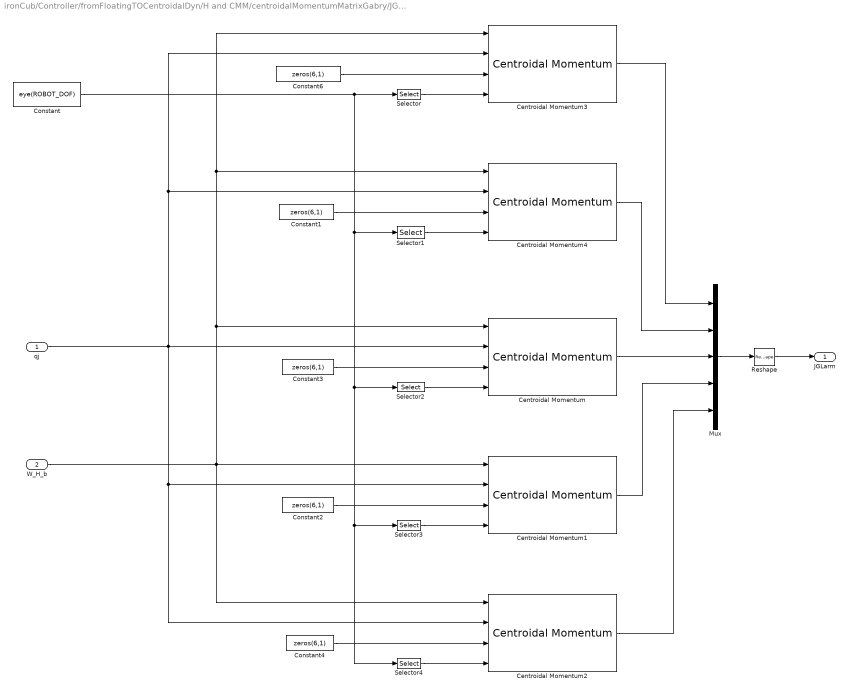
== system ironCub/Controller/fromFloatingTOCentroidalDyn/H and CMM/centroidalMomentumMatrixGabry/JGjoints/JGLarm ==
  qj : Inport
  W_H_b : Inport  Port=2
  Centroidal Momentum{,1..4} (5 alike) : WBToolboxLibrary/wholeBodyModel/Dynamics/Centroidal Momentum  robotName=WBT_robotName  localName=WBT_modelName  wbiFile=WBT_wbiFilename  wbiList=WBT_wbiList
  Constant : Constant  Value=eye(ROBOT_DOF)
  Constant{1..4,6} (5 alike) : Constant  Value=zeros(6,1)
  Mux : Mux  Inputs=5
  Reshape : Reshape  OutputDimensionality=Customize  OutputDimensions=[6,5]
  Selector : Selector  NumberOfDimensions=2  InputPortWidth=3  IndexOptions=Index vector (dialog),Select all  Indices=[4],1  OutputSizes=1,1
  Selector1 : Selector  NumberOfDimensions=2  InputPortWidth=3  IndexOptions=Index vector (dialog),Select all  Indices=[5],1  OutputSizes=1,1
  Selector2 : Selector  NumberOfDimensions=2  InputPortWidth=3  IndexOptions=Index vector (dialog),Select all  Indices=[6],1  OutputSizes=1,1
  Selector3 : Selector  NumberOfDimensions=2  InputPortWidth=3  IndexOptions=Index vector (dialog),Select all  Indices=[7],1  OutputSizes=1,1
  Selector4 : Selector  NumberOfDimensions=2  InputPortWidth=3  IndexOptions=Index vector (dialog),Select all  Indices=[8],1  OutputSizes=1,1
  JGLarm : Outport
  wires:
  Constant6/1 -> Centroidal Momentum3/3
  Constant1/1 -> Centroidal Momentum4/3
  Constant3/1 -> Centroidal Momentum/3
  Constant4/1 -> Centroidal Momentum2/3
  Constant2/1 -> Centroidal Momentum1/3
  qj/1 -> Centroidal Momentum4/2, Centroidal Momentum3/2, Centroidal Momentum2/2, Centroidal Momentum1/2, Centroidal Momentum/2
  W_H_b/1 -> Centroidal Momentum1/1, Centroidal Momentum2/1, Centroidal Momentum/1, Centroidal Momentum3/1, Centroidal Momentum4/1
  Constant/1 -> Selector4/1, Selector3/1, Selector2/1, Selector1/1, Selector/1
  Selector/1 -> Centroidal Momentum3/4
  Selector1/1 -> Centroidal Momentum4/4
  Selector2/1 -> Centroidal Momentum/4
  Selector3/1 -> Centroidal Momentum1/4
  Selector4/1 -> Centroidal Momentum2/4
  Centroidal Momentum/1 -> Mux/3
  Centroidal Momentum3/1 -> Mux/1
  Centroidal Momentum4/1 -> Mux/2
  Centroidal Momentum1/1 -> Mux/4
  Centroidal Momentum2/1 -> Mux/5
  Mux/1 -> Reshape/1
  Reshape/1 -> JGLarm/1

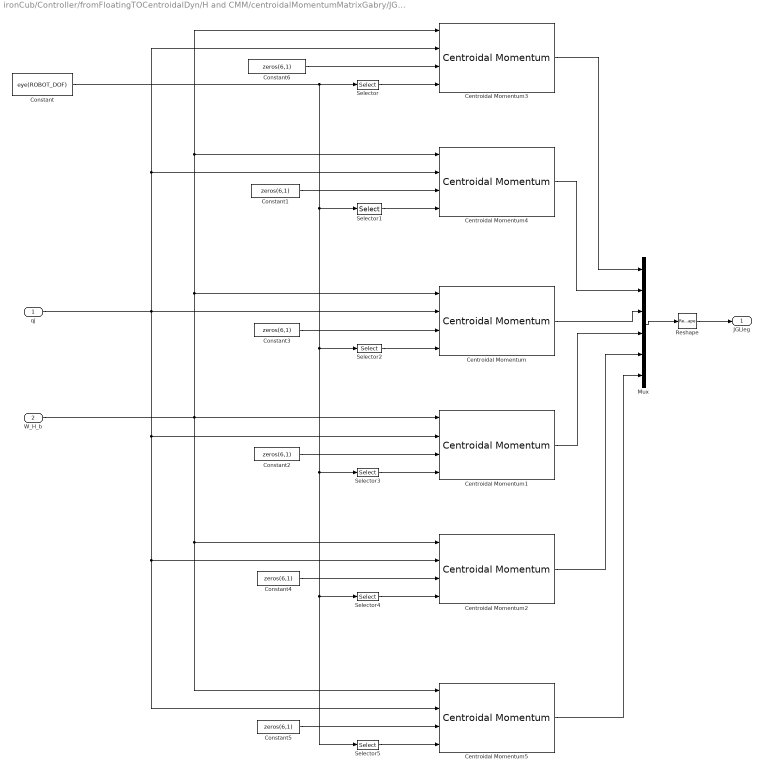
== system ironCub/Controller/fromFloatingTOCentroidalDyn/H and CMM/centroidalMomentumMatrixGabry/JGjoints/JGLleg ==
  qj : Inport
  W_H_b : Inport  Port=2
  Centroidal Momentum{,1..5} (6 alike) : WBToolboxLibrary/wholeBodyModel/Dynamics/Centroidal Momentum  robotName=WBT_robotName  localName=WBT_modelName  wbiFile=WBT_wbiFilename  wbiList=WBT_wbiList
  Constant : Constant  Value=eye(ROBOT_DOF)
  Constant{1..6} (6 alike) : Constant  Value=zeros(6,1)
  Mux : Mux  Inputs=6
  Reshape : Reshape  OutputDimensionality=Customize  OutputDimensions=[6,6]
  Selector : Selector  NumberOfDimensions=2  InputPortWidth=3  IndexOptions=Index vector (dialog),Select all  Indices=[14],1  OutputSizes=1,1
  Selector1 : Selector  NumberOfDimensions=2  InputPortWidth=3  IndexOptions=Index vector (dialog),Select all  Indices=[15],1  OutputSizes=1,1
  Selector2 : Selector  NumberOfDimensions=2  InputPortWidth=3  IndexOptions=Index vector (dialog),Select all  Indices=[16],1  OutputSizes=1,1
  Selector3 : Selector  NumberOfDimensions=2  InputPortWidth=3  IndexOptions=Index vector (dialog),Select all  Indices=[17],1  OutputSizes=1,1
  Selector4 : Selector  NumberOfDimensions=2  InputPortWidth=3  IndexOptions=Index vector (dialog),Select all  Indices=[18],1  OutputSizes=1,1
  Selector5 : Selector  NumberOfDimensions=2  InputPortWidth=3  IndexOptions=Index vector (dialog),Select all  Indices=[19],1  OutputSizes=1,1
  JGLleg : Outport
  wires:
  Constant6/1 -> Centroidal Momentum3/3
  Constant1/1 -> Centroidal Momentum4/3
  Constant3/1 -> Centroidal Momentum/3
  Constant4/1 -> Centroidal Momentum2/3
  Constant2/1 -> Centroidal Momentum1/3
  qj/1 -> Centroidal Momentum4/2, Centroidal Momentum3/2, Centroidal Momentum5/2, Centroidal Momentum2/2, Centroidal Momentum1/2, Centroidal Momentum/2
  W_H_b/1 -> Centroidal Momentum1/1, Centroidal Momentum5/1, Centroidal Momentum2/1, Centroidal Momentum/1, Centroidal Momentum3/1, Centroidal Momentum4/1
  Selector/1 -> Centroidal Momentum3/4
  Selector1/1 -> Centroidal Momentum4/4
  Selector2/1 -> Centroidal Momentum/4
  Selector3/1 -> Centroidal Momentum1/4
  Selector4/1 -> Centroidal Momentum2/4
  Centroidal Momentum/1 -> Mux/3
  Centroidal Momentum3/1 -> Mux/1
  Centroidal Momentum4/1 -> Mux/2
  Centroidal Momentum1/1 -> Mux/4
  Centroidal Momentum2/1 -> Mux/5
  Mux/1 -> Reshape/1
  Reshape/1 -> JGLleg/1
  Constant5/1 -> Centroidal Momentum5/3
  Constant/1 -> Selector5/1, Selector4/1, Selector3/1, Selector2/1, Selector1/1, Selector/1
  Selector5/1 -> Centroidal Momentum5/4
  Centroidal Momentum5/1 -> Mux/6
